simulink model "optimal_dosing"  (R2020a)
settings: Solver=VariableStepAuto  StartTime=0.0  StopTime=15  RelTol=1e-3
values from neighbouring files (symbols this model uses):
  circ0 = 5.04    [project3.m]
  Edrugss = Edrugf    (= 0.176268421044)    [project3.m]
  Fopt = lqr(A,B,R1,R2)    [project3.m]
  gamma = 0.16    [project3.m]
  kcirc = 4/120.4    (= 0.0332225913621)    [project3.m]
  ktr = 4/120.4    (= 0.0332225913621)    [project3.m]
  x1ss = ANC    (= 1.5)    [project3.m]
  x2ss = circ0    (= 5.04)    [project3.m]
  x3ss = circ0    (= 5.04)    [project3.m]
  x4ss = circ0    (= 5.04)    [project3.m]
  x5ss = circ0    (= 5.04)    [project3.m]
settings Model: Creator=Alan  LastModifiedBy=Alan

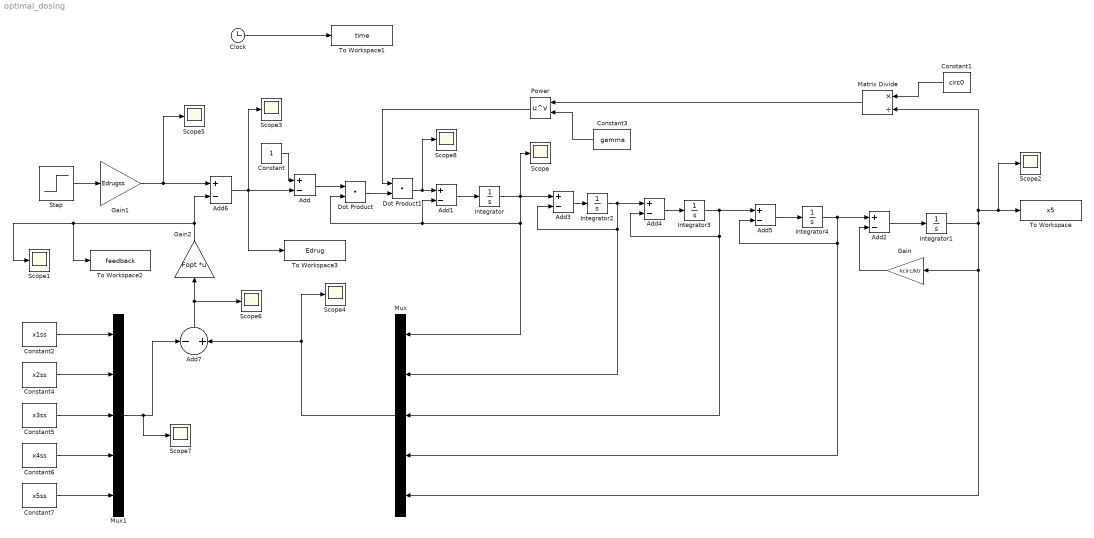
== system optimal_dosing ==
  Add{,1..6} (7 alike) : Sum  Inputs=+-
  Add7 : Sum  Inputs=-+
  Clock : Clock
  Constant : Constant
  Constant1 : Constant  Value=circ0
  Constant2 : Constant  Value=x1ss
  Constant3 : Constant  Value=gamma
  Constant4 : Constant  Value=x2ss
  Constant5 : Constant  Value=x3ss
  Constant6 : Constant  Value=x4ss
  Constant7 : Constant  Value=x5ss
  Dot Product : DotProduct  OutDataTypeStr=Inherit: Inherit via internal rule
  Dot Product1 : DotProduct  OutDataTypeStr=Inherit: Inherit via internal rule
  Gain : Gain  Gain=kcirc/ktr
  Gain1 : Gain  Gain=Edrugss
  Gain2 : Gain  Gain=Fopt  Multiplication=Matrix(K*u)
  Integrator : Integrator  InitialCondition=x1ss
  Integrator1 : Integrator  InitialCondition=x5ss
  Integrator2 : Integrator  InitialCondition=x2ss
  Integrator3 : Integrator  InitialCondition=x3ss
  Integrator4 : Integrator  InitialCondition=x4ss
  Matrix Divide : Product  Inputs=*/
  Mux : Mux  Inputs=5
  Mux1 : Mux  Inputs=5
  Power : Math  Operator=pow  SaturateOnIntegerOverflow=on
  Scope{,1..8} (9 alike) : Scope
  Step : Step  Time=0  SampleTime=0
  To Workspace : ToWorkspace  VariableName=x5  SampleTime=-1
  To Workspace1 : ToWorkspace  VariableName=time  SampleTime=-1
  To Workspace2 : ToWorkspace  VariableName=feedback  SampleTime=-1
  To Workspace3 : ToWorkspace  VariableName=Edrug  SampleTime=-1
  wires:
  Integrator/1 -> Add3/1, Scope/1, Mux/1, Dot Product/2, Add1/2
  Dot Product1/1 -> Scope8/1, Add1/1
  Add2/1 -> Integrator1/1
  Add1/1 -> Integrator/1
  Integrator1/1 -> Mux/5, Gain/1, Matrix Divide/2, Scope2/1, To Workspace/1
  Gain/1 -> Add2/2
  Power/1 -> Dot Product1/1
  Constant1/1 -> Matrix Divide/1
  Clock/1 -> To Workspace1/1
  Dot Product/1 -> Dot Product1/2
  Constant3/1 -> Power/2
  Add/1 -> Dot Product/1
  Constant/1 -> Add/1
  Matrix Divide/1 -> Power/1
  Integrator4/1 -> Add2/1, Mux/4, Add5/2
  Add3/1 -> Integrator2/1
  Add4/1 -> Integrator3/1
  Add5/1 -> Integrator4/1
  Integrator2/1 -> Add4/1, Add3/2, Mux/2
  Integrator3/1 -> Add5/1, Mux/3, Add4/2
  Gain1/1 -> Scope5/1, Add6/1
  Add6/1 -> To Workspace3/1, Add/2, Scope3/1
  Step/1 -> Gain1/1
  Mux1/1 -> Scope7/1, Add7/1
  Mux/1 -> Add7/2, Scope4/1
  Add7/1 -> Gain2/1, Scope6/1
  Gain2/1 -> To Workspace2/1, Scope1/1, Add6/2
  Constant2/1 -> Mux1/1
  Constant4/1 -> Mux1/2
  Constant5/1 -> Mux1/3
  Constant6/1 -> Mux1/4
  Constant7/1 -> Mux1/5
